simulink model "calculate_k11"  (R2022b)
settings: Solver=VariableStepAuto  StartTime=0.0  StopTime=10.0  RelTol=1e-3
values from neighbouring files (symbols this model uses):
  k1 = 0.624    [run_first.m]
  k2 = -0.015    [run_first.m]
  k3 = -0.0006    [run_first.m]
settings Model: Creator=fabian  LastModifiedBy=fabian

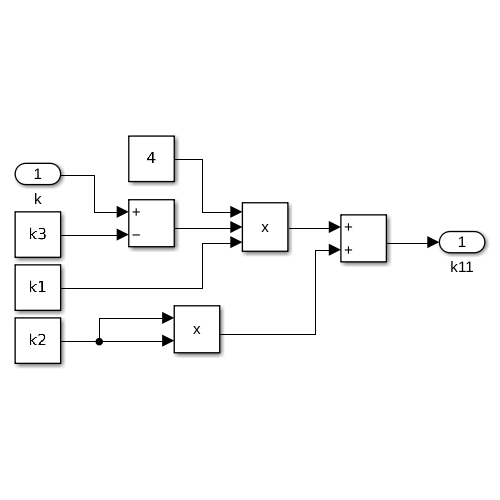
[thumbnail: Simulink's stored preview of the top-level diagram]
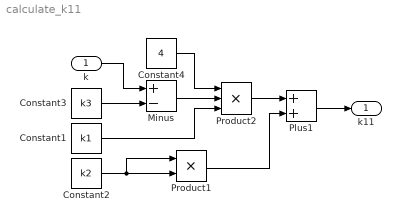
== system calculate_k11 ==
  k : Inport
  Constant1 : Constant  Value=k1
  Constant2 : Constant  Value=k2
  Constant3 : Constant  Value=k3
  Constant4 : Constant  Value=4
  Minus : Sum  Inputs=+-
  Plus1 : Sum
  Product1 : Product
  Product2 : Product  Inputs=3
  k11 : Outport
  wires:
  Minus/1 -> Product2/2
  Product2/1 -> Plus1/1
  Constant2/1 -> Product1/1, Product1/2
  Constant3/1 -> Minus/2
  Product1/1 -> Plus1/2
  Constant1/1 -> Product2/3
  Constant4/1 -> Product2/1
  k/1 -> Minus/1
  Plus1/1 -> k11/1
